simulink library "HvsOpen"  (Simulink 7.8)
settings: Solver=ode45  StartTime=0.0  StopTime=10.0  RelTol=1e-3
(part 1 of 2)
settings Model: Creator=KLJS168  LastModifiedBy=KLJS168

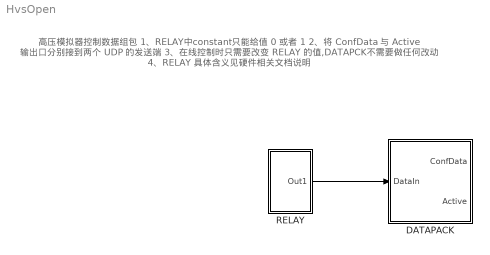
== system HvsOpen ==
  note: 高压模拟器控制数据组包
      | 1、RELAY中constant只能给值 0 或者 1
      | 2、将 ConfData 与 Active 输出口分别接到两个 UDP 的发送端
      | 3、在线控制时只需要改变 RELAY 的值,DATAPCK不需要做任何改动
      | 4、RELAY 具体含义见硬件相关文档说明
  DATAPACK : Subsystem
  RELAY : Subsystem
  wires:
  RELAY/1(Out1) -> DATAPACK/1(DataIn)

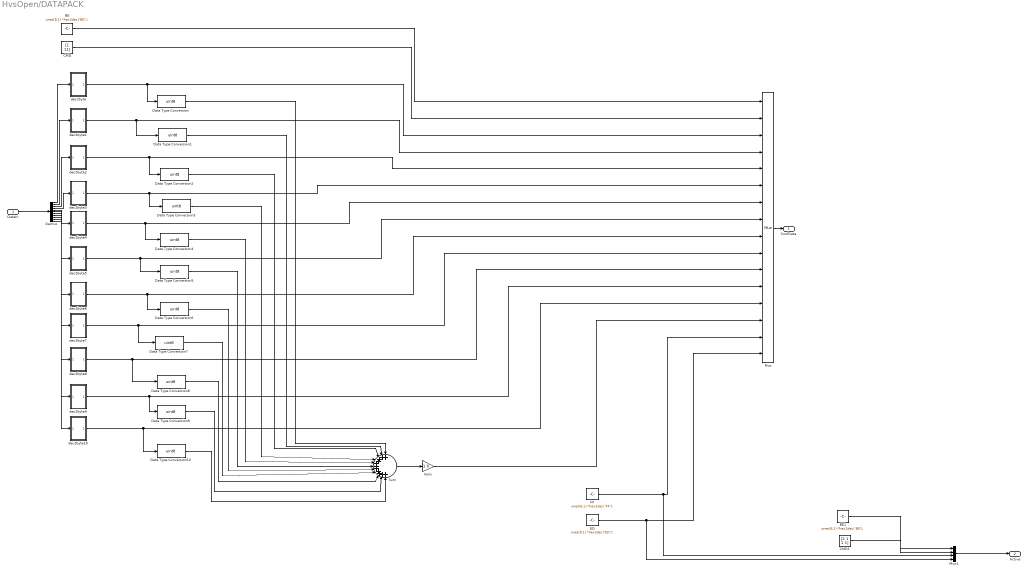
== system HvsOpen/DATAPACK ==
  DataIn : Inport
  BE : Constant  Value=ones(8,1).*hex2dec('BE');
  BE1 : Constant  Value=ones(8,1).*hex2dec('BE');
  CMD : Constant  Value=[1 11]
  CMD1 : Constant  Value=[2 1 1 1]
  Data Type Conversion{,1..10} (11 alike) : DataTypeConversion  OutDataTypeStr=uint8
  Demux : Demux  Outputs=[8 8 8 8 8 8 8 8 8 8 8]
  ED : Constant  Value=ones(8,1).*hex2dec('ED');
  FF : Constant  Value=ones(8,1).*hex2dec('FF');
  Gain : Gain  Gain=1.0  OutDataTypeStr=double
  Mux : Mux  Inputs=[8 2 1 1 1 1 1 1 1 1 1 1 1 1 8 8]
  Mux1 : Mux  Inputs=[8 4 8 8]
  Sum : Sum  Inputs=+++++++++++
  dec2byte : Subsystem
  dec2byte1 : Subsystem
  dec2byte10 : Subsystem
  dec2byte2 : Subsystem
  dec2byte3 : Subsystem
  dec2byte4 : Subsystem
  dec2byte5 : Subsystem
  dec2byte6 : Subsystem
  dec2byte7 : Subsystem
  dec2byte8 : Subsystem
  dec2byte9 : Subsystem
  ConfData : Outport
  Active : Outport  Port=2
  wires:
  BE/1 -> Mux/1
  CMD/1 -> Mux/2
  dec2byte/1(Out1) -> Mux/3, Data Type Conversion/1
  dec2byte1/1(Out1) -> Mux/4, Data Type Conversion1/1
  dec2byte2/1(Out1) -> Mux/5, Data Type Conversion2/1
  dec2byte3/1(Out1) -> Mux/6, Data Type Conversion3/1
  dec2byte4/1(Out1) -> Mux/7, Data Type Conversion4/1
  dec2byte5/1(Out1) -> Mux/8, Data Type Conversion5/1
  dec2byte6/1(Out1) -> Mux/9, Data Type Conversion6/1
  dec2byte7/1(Out1) -> Mux/10, Data Type Conversion7/1
  dec2byte8/1(Out1) -> Mux/11, Data Type Conversion8/1
  dec2byte9/1(Out1) -> Mux/12, Data Type Conversion9/1
  dec2byte10/1(Out1) -> Mux/13, Data Type Conversion10/1
  Sum/1 -> Gain/1
  Gain/1 -> Mux/14
  FF/1 -> Mux/15, Mux1/3
  ED/1 -> Mux/16, Mux1/4
  Data Type Conversion/1 -> Sum/1
  Data Type Conversion1/1 -> Sum/2
  Data Type Conversion2/1 -> Sum/3
  Data Type Conversion3/1 -> Sum/4
  Data Type Conversion4/1 -> Sum/5
  Data Type Conversion5/1 -> Sum/6
  Data Type Conversion6/1 -> Sum/7
  Data Type Conversion7/1 -> Sum/8
  Data Type Conversion8/1 -> Sum/9
  Data Type Conversion9/1 -> Sum/10
  Data Type Conversion10/1 -> Sum/11
  Mux/1 -> ConfData/1
  Demux/1 -> dec2byte/1(In1)
  Demux/2 -> dec2byte1/1(In1)
  Demux/3 -> dec2byte2/1(In1)
  Demux/4 -> dec2byte3/1(In1)
  Demux/5 -> dec2byte4/1(In1)
  Demux/6 -> dec2byte5/1(In1)
  Demux/7 -> dec2byte6/1(In1)
  Demux/8 -> dec2byte7/1(In1)
  Demux/9 -> dec2byte8/1(In1)
  Demux/10 -> dec2byte9/1(In1)
  Demux/11 -> dec2byte10/1(In1)
  DataIn/1 -> Demux/1
  BE1/1 -> Mux1/1
  CMD1/1 -> Mux1/2
  Mux1/1 -> Active/1

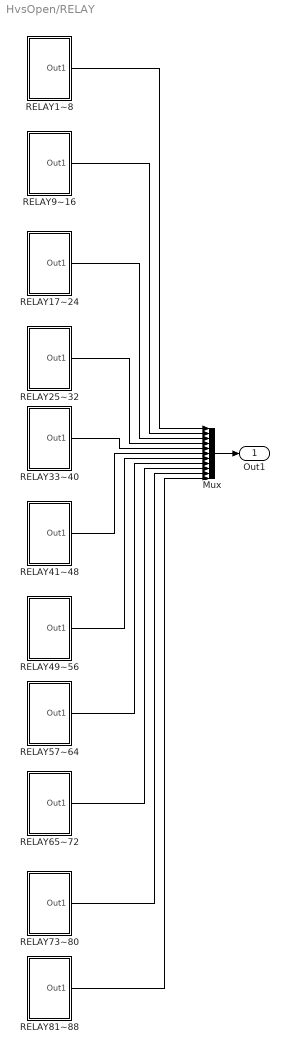
== system HvsOpen/RELAY ==
  Mux : Mux  Inputs=[8 8 8 8 8 8 8 8 8 8 8]
  RELAY17~24 : Subsystem
  RELAY1~8 : Subsystem
  RELAY25~32 : Subsystem
  RELAY33~40 : Subsystem
  RELAY41~48 : Subsystem
  RELAY49~56 : Subsystem
  RELAY57~64 : Subsystem
  RELAY65~72 : Subsystem
  RELAY73~80 : Subsystem
  RELAY81~88 : Subsystem
  RELAY9~16 : Subsystem
  Out1 : Outport
  wires:
  RELAY1~8/1(Out1) -> Mux/1
  RELAY9~16/1(Out1) -> Mux/2
  RELAY17~24/1(Out1) -> Mux/3
  RELAY25~32/1(Out1) -> Mux/4
  RELAY33~40/1(Out1) -> Mux/5
  RELAY41~48/1(Out1) -> Mux/6
  RELAY49~56/1(Out1) -> Mux/7
  RELAY57~64/1(Out1) -> Mux/8
  RELAY65~72/1(Out1) -> Mux/9
  RELAY73~80/1(Out1) -> Mux/10
  RELAY81~88/1(Out1) -> Mux/11
  Mux/1 -> Out1/1

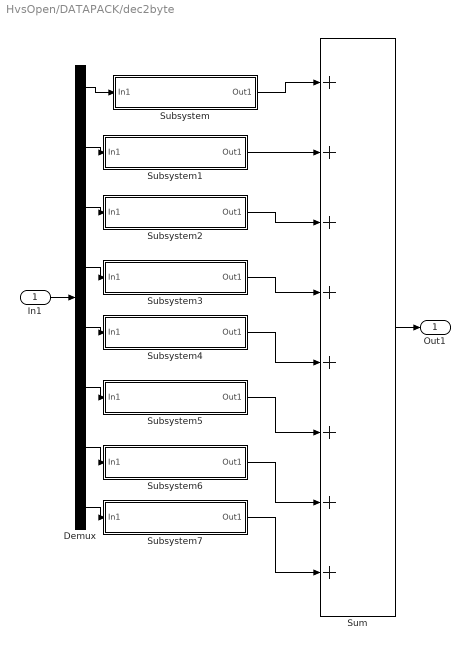
== system HvsOpen/DATAPACK/dec2byte ==
  In1 : Inport
  Demux : Demux  Outputs=8
  Subsystem : Subsystem  mask{power=0}
  Subsystem1 : Subsystem  mask{power=1}
  Subsystem2 : Subsystem  mask{power=2}
  Subsystem3 : Subsystem  mask{power=3}
  Subsystem4 : Subsystem  mask{power=4}
  Subsystem5 : Subsystem  mask{power=5}
  Subsystem6 : Subsystem  mask{power=6}
  Subsystem7 : Subsystem  mask{power=7}
  Sum : Sum  Inputs=++++++++
  Out1 : Outport
  wires:
  Demux/1 -> Subsystem/1(In1)
  Demux/2 -> Subsystem1/1(In1)
  Demux/3 -> Subsystem2/1(In1)
  Demux/4 -> Subsystem3/1(In1)
  Demux/5 -> Subsystem4/1(In1)
  Demux/6 -> Subsystem5/1(In1)
  Demux/7 -> Subsystem6/1(In1)
  Demux/8 -> Subsystem7/1(In1)
  Subsystem/1(Out1) -> Sum/1
  Subsystem1/1(Out1) -> Sum/2
  Subsystem2/1(Out1) -> Sum/3
  Subsystem3/1(Out1) -> Sum/4
  Subsystem4/1(Out1) -> Sum/5
  Subsystem5/1(Out1) -> Sum/6
  Subsystem6/1(Out1) -> Sum/7
  Subsystem7/1(Out1) -> Sum/8
  In1/1 -> Demux/1
  Sum/1 -> Out1/1

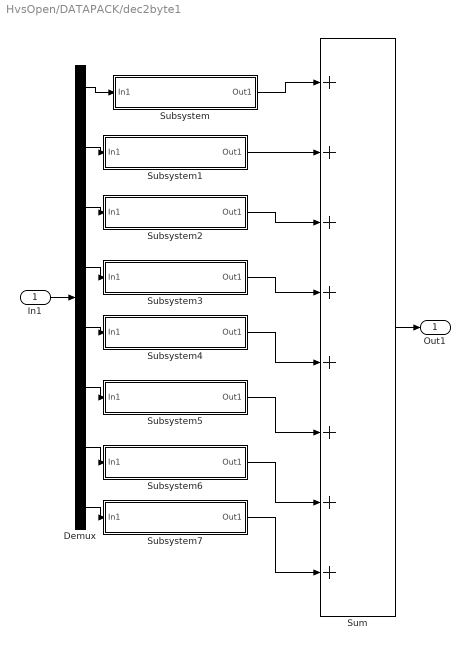
== system HvsOpen/DATAPACK/dec2byte1 ==
  In1 : Inport
  Demux : Demux  Outputs=8
  Subsystem : Subsystem  mask{power=0}
  Subsystem1 : Subsystem  mask{power=1}
  Subsystem2 : Subsystem  mask{power=2}
  Subsystem3 : Subsystem  mask{power=3}
  Subsystem4 : Subsystem  mask{power=4}
  Subsystem5 : Subsystem  mask{power=5}
  Subsystem6 : Subsystem  mask{power=6}
  Subsystem7 : Subsystem  mask{power=7}
  Sum : Sum  Inputs=++++++++
  Out1 : Outport
  wires:
  Sum/1 -> Out1/1
  In1/1 -> Demux/1
  Subsystem7/1(Out1) -> Sum/8
  Subsystem6/1(Out1) -> Sum/7
  Subsystem5/1(Out1) -> Sum/6
  Subsystem4/1(Out1) -> Sum/5
  Subsystem3/1(Out1) -> Sum/4
  Subsystem2/1(Out1) -> Sum/3
  Subsystem1/1(Out1) -> Sum/2
  Subsystem/1(Out1) -> Sum/1
  Demux/8 -> Subsystem7/1(In1)
  Demux/7 -> Subsystem6/1(In1)
  Demux/6 -> Subsystem5/1(In1)
  Demux/5 -> Subsystem4/1(In1)
  Demux/4 -> Subsystem3/1(In1)
  Demux/3 -> Subsystem2/1(In1)
  Demux/2 -> Subsystem1/1(In1)
  Demux/1 -> Subsystem/1(In1)

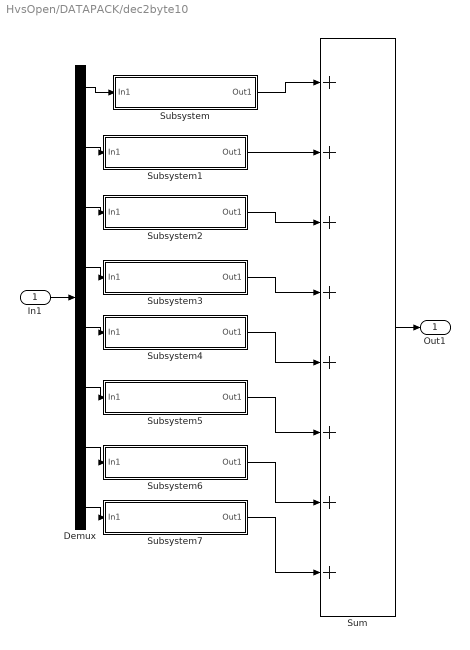
== system HvsOpen/DATAPACK/dec2byte10 ==
  In1 : Inport
  Demux : Demux  Outputs=8
  Subsystem : Subsystem  mask{power=0}
  Subsystem1 : Subsystem  mask{power=1}
  Subsystem2 : Subsystem  mask{power=2}
  Subsystem3 : Subsystem  mask{power=3}
  Subsystem4 : Subsystem  mask{power=4}
  Subsystem5 : Subsystem  mask{power=5}
  Subsystem6 : Subsystem  mask{power=6}
  Subsystem7 : Subsystem  mask{power=7}
  Sum : Sum  Inputs=++++++++
  Out1 : Outport
  wires:
  Demux/1 -> Subsystem/1(In1)
  Demux/2 -> Subsystem1/1(In1)
  Demux/3 -> Subsystem2/1(In1)
  Demux/4 -> Subsystem3/1(In1)
  Demux/5 -> Subsystem4/1(In1)
  Demux/6 -> Subsystem5/1(In1)
  Demux/7 -> Subsystem6/1(In1)
  Demux/8 -> Subsystem7/1(In1)
  Subsystem/1(Out1) -> Sum/1
  Subsystem1/1(Out1) -> Sum/2
  Subsystem2/1(Out1) -> Sum/3
  Subsystem3/1(Out1) -> Sum/4
  Subsystem4/1(Out1) -> Sum/5
  Subsystem5/1(Out1) -> Sum/6
  Subsystem6/1(Out1) -> Sum/7
  Subsystem7/1(Out1) -> Sum/8
  In1/1 -> Demux/1
  Sum/1 -> Out1/1

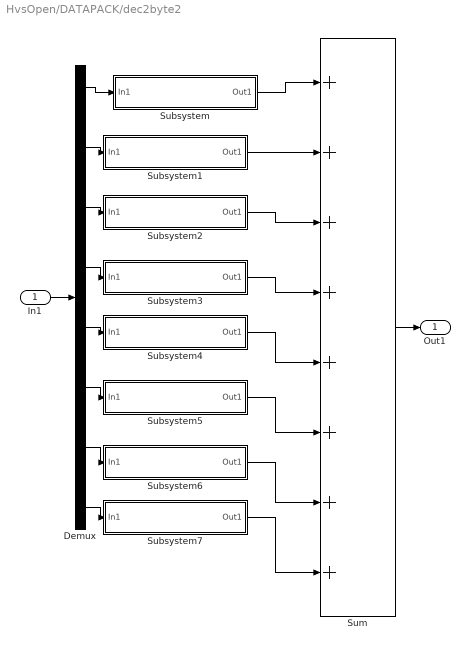
== system HvsOpen/DATAPACK/dec2byte2 ==
  In1 : Inport
  Demux : Demux  Outputs=8
  Subsystem : Subsystem  mask{power=0}
  Subsystem1 : Subsystem  mask{power=1}
  Subsystem2 : Subsystem  mask{power=2}
  Subsystem3 : Subsystem  mask{power=3}
  Subsystem4 : Subsystem  mask{power=4}
  Subsystem5 : Subsystem  mask{power=5}
  Subsystem6 : Subsystem  mask{power=6}
  Subsystem7 : Subsystem  mask{power=7}
  Sum : Sum  Inputs=++++++++
  Out1 : Outport
  wires:
  Demux/1 -> Subsystem/1(In1)
  Demux/2 -> Subsystem1/1(In1)
  Demux/3 -> Subsystem2/1(In1)
  Demux/4 -> Subsystem3/1(In1)
  Demux/5 -> Subsystem4/1(In1)
  Demux/6 -> Subsystem5/1(In1)
  Demux/7 -> Subsystem6/1(In1)
  Demux/8 -> Subsystem7/1(In1)
  Subsystem/1(Out1) -> Sum/1
  Subsystem1/1(Out1) -> Sum/2
  Subsystem2/1(Out1) -> Sum/3
  Subsystem3/1(Out1) -> Sum/4
  Subsystem4/1(Out1) -> Sum/5
  Subsystem5/1(Out1) -> Sum/6
  Subsystem6/1(Out1) -> Sum/7
  Subsystem7/1(Out1) -> Sum/8
  In1/1 -> Demux/1
  Sum/1 -> Out1/1

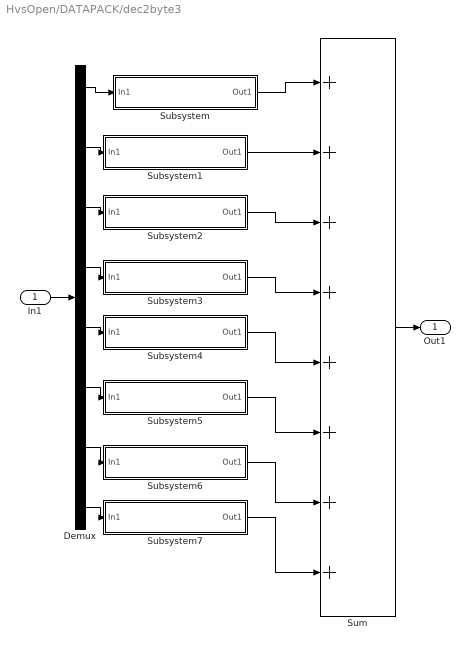
== system HvsOpen/DATAPACK/dec2byte3 ==
  In1 : Inport
  Demux : Demux  Outputs=8
  Subsystem : Subsystem  mask{power=0}
  Subsystem1 : Subsystem  mask{power=1}
  Subsystem2 : Subsystem  mask{power=2}
  Subsystem3 : Subsystem  mask{power=3}
  Subsystem4 : Subsystem  mask{power=4}
  Subsystem5 : Subsystem  mask{power=5}
  Subsystem6 : Subsystem  mask{power=6}
  Subsystem7 : Subsystem  mask{power=7}
  Sum : Sum  Inputs=++++++++
  Out1 : Outport
  wires:
  Sum/1 -> Out1/1
  In1/1 -> Demux/1
  Subsystem7/1(Out1) -> Sum/8
  Subsystem6/1(Out1) -> Sum/7
  Subsystem5/1(Out1) -> Sum/6
  Subsystem4/1(Out1) -> Sum/5
  Subsystem3/1(Out1) -> Sum/4
  Subsystem2/1(Out1) -> Sum/3
  Subsystem1/1(Out1) -> Sum/2
  Subsystem/1(Out1) -> Sum/1
  Demux/8 -> Subsystem7/1(In1)
  Demux/7 -> Subsystem6/1(In1)
  Demux/6 -> Subsystem5/1(In1)
  Demux/5 -> Subsystem4/1(In1)
  Demux/4 -> Subsystem3/1(In1)
  Demux/3 -> Subsystem2/1(In1)
  Demux/2 -> Subsystem1/1(In1)
  Demux/1 -> Subsystem/1(In1)

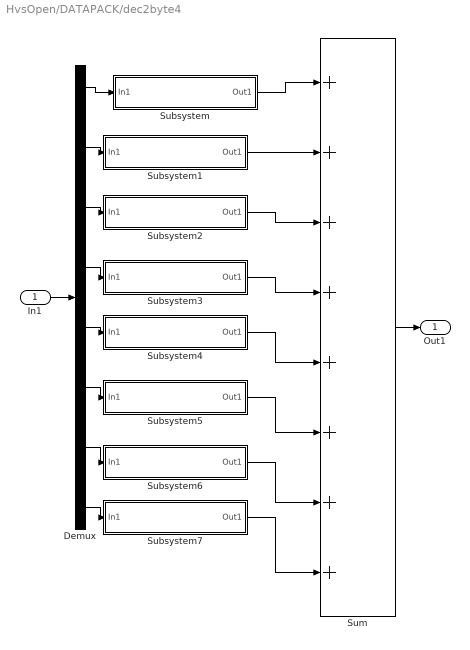
== system HvsOpen/DATAPACK/dec2byte4 ==
  In1 : Inport
  Demux : Demux  Outputs=8
  Subsystem : Subsystem  mask{power=0}
  Subsystem1 : Subsystem  mask{power=1}
  Subsystem2 : Subsystem  mask{power=2}
  Subsystem3 : Subsystem  mask{power=3}
  Subsystem4 : Subsystem  mask{power=4}
  Subsystem5 : Subsystem  mask{power=5}
  Subsystem6 : Subsystem  mask{power=6}
  Subsystem7 : Subsystem  mask{power=7}
  Sum : Sum  Inputs=++++++++
  Out1 : Outport
  wires:
  Demux/1 -> Subsystem/1(In1)
  Demux/2 -> Subsystem1/1(In1)
  Demux/3 -> Subsystem2/1(In1)
  Demux/4 -> Subsystem3/1(In1)
  Demux/5 -> Subsystem4/1(In1)
  Demux/6 -> Subsystem5/1(In1)
  Demux/7 -> Subsystem6/1(In1)
  Demux/8 -> Subsystem7/1(In1)
  Subsystem/1(Out1) -> Sum/1
  Subsystem1/1(Out1) -> Sum/2
  Subsystem2/1(Out1) -> Sum/3
  Subsystem3/1(Out1) -> Sum/4
  Subsystem4/1(Out1) -> Sum/5
  Subsystem5/1(Out1) -> Sum/6
  Subsystem6/1(Out1) -> Sum/7
  Subsystem7/1(Out1) -> Sum/8
  In1/1 -> Demux/1
  Sum/1 -> Out1/1

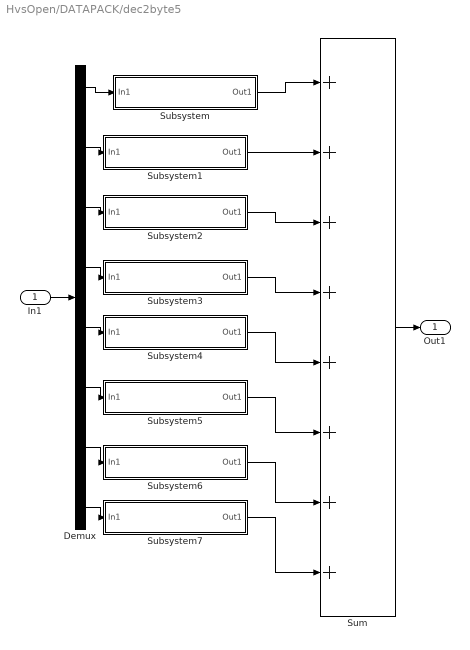
== system HvsOpen/DATAPACK/dec2byte5 ==
  In1 : Inport
  Demux : Demux  Outputs=8
  Subsystem : Subsystem  mask{power=0}
  Subsystem1 : Subsystem  mask{power=1}
  Subsystem2 : Subsystem  mask{power=2}
  Subsystem3 : Subsystem  mask{power=3}
  Subsystem4 : Subsystem  mask{power=4}
  Subsystem5 : Subsystem  mask{power=5}
  Subsystem6 : Subsystem  mask{power=6}
  Subsystem7 : Subsystem  mask{power=7}
  Sum : Sum  Inputs=++++++++
  Out1 : Outport
  wires:
  Sum/1 -> Out1/1
  In1/1 -> Demux/1
  Subsystem7/1(Out1) -> Sum/8
  Subsystem6/1(Out1) -> Sum/7
  Subsystem5/1(Out1) -> Sum/6
  Subsystem4/1(Out1) -> Sum/5
  Subsystem3/1(Out1) -> Sum/4
  Subsystem2/1(Out1) -> Sum/3
  Subsystem1/1(Out1) -> Sum/2
  Subsystem/1(Out1) -> Sum/1
  Demux/8 -> Subsystem7/1(In1)
  Demux/7 -> Subsystem6/1(In1)
  Demux/6 -> Subsystem5/1(In1)
  Demux/5 -> Subsystem4/1(In1)
  Demux/4 -> Subsystem3/1(In1)
  Demux/3 -> Subsystem2/1(In1)
  Demux/2 -> Subsystem1/1(In1)
  Demux/1 -> Subsystem/1(In1)

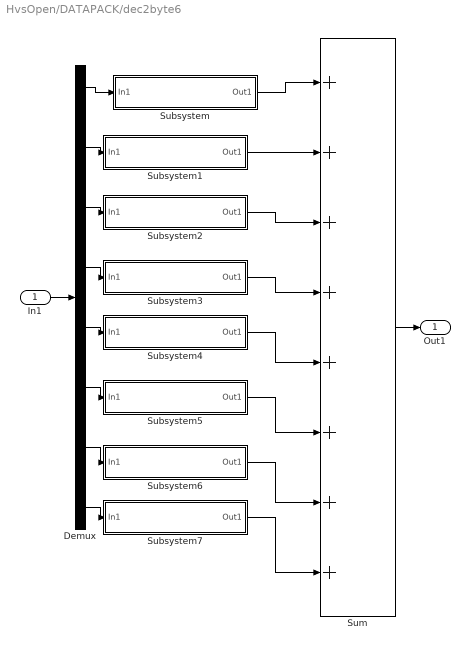
== system HvsOpen/DATAPACK/dec2byte6 ==
  In1 : Inport
  Demux : Demux  Outputs=8
  Subsystem : Subsystem  mask{power=0}
  Subsystem1 : Subsystem  mask{power=1}
  Subsystem2 : Subsystem  mask{power=2}
  Subsystem3 : Subsystem  mask{power=3}
  Subsystem4 : Subsystem  mask{power=4}
  Subsystem5 : Subsystem  mask{power=5}
  Subsystem6 : Subsystem  mask{power=6}
  Subsystem7 : Subsystem  mask{power=7}
  Sum : Sum  Inputs=++++++++
  Out1 : Outport
  wires:
  Demux/1 -> Subsystem/1(In1)
  Demux/2 -> Subsystem1/1(In1)
  Demux/3 -> Subsystem2/1(In1)
  Demux/4 -> Subsystem3/1(In1)
  Demux/5 -> Subsystem4/1(In1)
  Demux/6 -> Subsystem5/1(In1)
  Demux/7 -> Subsystem6/1(In1)
  Demux/8 -> Subsystem7/1(In1)
  Subsystem/1(Out1) -> Sum/1
  Subsystem1/1(Out1) -> Sum/2
  Subsystem2/1(Out1) -> Sum/3
  Subsystem3/1(Out1) -> Sum/4
  Subsystem4/1(Out1) -> Sum/5
  Subsystem5/1(Out1) -> Sum/6
  Subsystem6/1(Out1) -> Sum/7
  Subsystem7/1(Out1) -> Sum/8
  In1/1 -> Demux/1
  Sum/1 -> Out1/1

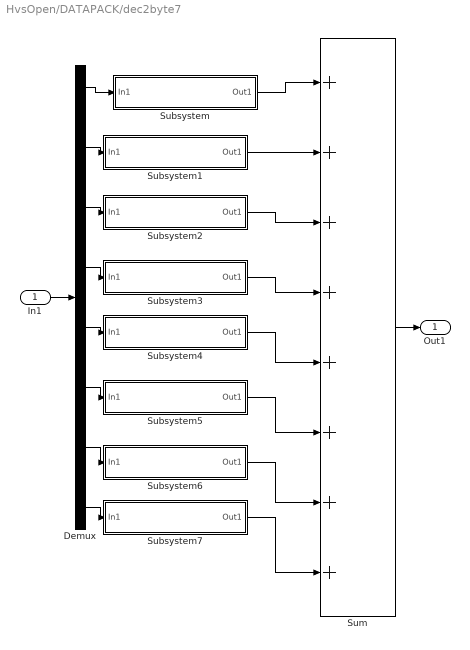
== system HvsOpen/DATAPACK/dec2byte7 ==
  In1 : Inport
  Demux : Demux  Outputs=8
  Subsystem : Subsystem  mask{power=0}
  Subsystem1 : Subsystem  mask{power=1}
  Subsystem2 : Subsystem  mask{power=2}
  Subsystem3 : Subsystem  mask{power=3}
  Subsystem4 : Subsystem  mask{power=4}
  Subsystem5 : Subsystem  mask{power=5}
  Subsystem6 : Subsystem  mask{power=6}
  Subsystem7 : Subsystem  mask{power=7}
  Sum : Sum  Inputs=++++++++
  Out1 : Outport
  wires:
  Sum/1 -> Out1/1
  In1/1 -> Demux/1
  Subsystem7/1(Out1) -> Sum/8
  Subsystem6/1(Out1) -> Sum/7
  Subsystem5/1(Out1) -> Sum/6
  Subsystem4/1(Out1) -> Sum/5
  Subsystem3/1(Out1) -> Sum/4
  Subsystem2/1(Out1) -> Sum/3
  Subsystem1/1(Out1) -> Sum/2
  Subsystem/1(Out1) -> Sum/1
  Demux/8 -> Subsystem7/1(In1)
  Demux/7 -> Subsystem6/1(In1)
  Demux/6 -> Subsystem5/1(In1)
  Demux/5 -> Subsystem4/1(In1)
  Demux/4 -> Subsystem3/1(In1)
  Demux/3 -> Subsystem2/1(In1)
  Demux/2 -> Subsystem1/1(In1)
  Demux/1 -> Subsystem/1(In1)

== system HvsOpen/DATAPACK/dec2byte8 ==
  In1 : Inport
  Demux : Demux  Outputs=8
  Subsystem : Subsystem  mask{power=0}
  Subsystem1 : Subsystem  mask{power=1}
  Subsystem2 : Subsystem  mask{power=2}
  Subsystem3 : Subsystem  mask{power=3}
  Subsystem4 : Subsystem  mask{power=4}
  Subsystem5 : Subsystem  mask{power=5}
  Subsystem6 : Subsystem  mask{power=6}
  Subsystem7 : Subsystem  mask{power=7}
  Sum : Sum  Inputs=++++++++
  Out1 : Outport
  wires:
  Demux/1 -> Subsystem/1(In1)
  Demux/2 -> Subsystem1/1(In1)
  Demux/3 -> Subsystem2/1(In1)
  Demux/4 -> Subsystem3/1(In1)
  Demux/5 -> Subsystem4/1(In1)
  Demux/6 -> Subsystem5/1(In1)
  Demux/7 -> Subsystem6/1(In1)
  Demux/8 -> Subsystem7/1(In1)
  Subsystem/1(Out1) -> Sum/1
  Subsystem1/1(Out1) -> Sum/2
  Subsystem2/1(Out1) -> Sum/3
  Subsystem3/1(Out1) -> Sum/4
  Subsystem4/1(Out1) -> Sum/5
  Subsystem5/1(Out1) -> Sum/6
  Subsystem6/1(Out1) -> Sum/7
  Subsystem7/1(Out1) -> Sum/8
  In1/1 -> Demux/1
  Sum/1 -> Out1/1

== system HvsOpen/DATAPACK/dec2byte9 ==
  In1 : Inport
  Demux : Demux  Outputs=8
  Subsystem : Subsystem  mask{power=0}
  Subsystem1 : Subsystem  mask{power=1}
  Subsystem2 : Subsystem  mask{power=2}
  Subsystem3 : Subsystem  mask{power=3}
  Subsystem4 : Subsystem  mask{power=4}
  Subsystem5 : Subsystem  mask{power=5}
  Subsystem6 : Subsystem  mask{power=6}
  Subsystem7 : Subsystem  mask{power=7}
  Sum : Sum  Inputs=++++++++
  Out1 : Outport
  wires:
  Sum/1 -> Out1/1
  In1/1 -> Demux/1
  Subsystem7/1(Out1) -> Sum/8
  Subsystem6/1(Out1) -> Sum/7
  Subsystem5/1(Out1) -> Sum/6
  Subsystem4/1(Out1) -> Sum/5
  Subsystem3/1(Out1) -> Sum/4
  Subsystem2/1(Out1) -> Sum/3
  Subsystem1/1(Out1) -> Sum/2
  Subsystem/1(Out1) -> Sum/1
  Demux/8 -> Subsystem7/1(In1)
  Demux/7 -> Subsystem6/1(In1)
  Demux/6 -> Subsystem5/1(In1)
  Demux/5 -> Subsystem4/1(In1)
  Demux/4 -> Subsystem3/1(In1)
  Demux/3 -> Subsystem2/1(In1)
  Demux/2 -> Subsystem1/1(In1)
  Demux/1 -> Subsystem/1(In1)

== system HvsOpen/RELAY/RELAY17~24 ==
  Mux : Mux  Inputs=8
  No USE : Constant  Value=0
  RELAY{18..24} (7 alike) : Constant  Value=0
  Out1 : Outport
  wires:
  Mux/1 -> Out1/1
  No USE/1 -> Mux/1
  RELAY18/1 -> Mux/2
  RELAY19/1 -> Mux/3
  RELAY20/1 -> Mux/4
  RELAY21/1 -> Mux/5
  RELAY22/1 -> Mux/6
  RELAY23/1 -> Mux/7
  RELAY24/1 -> Mux/8

== system HvsOpen/RELAY/RELAY1~8 ==
  Mux : Mux  Inputs=8
  RELAY{1..8} (8 alike) : Constant  Value=0
  Out1 : Outport
  wires:
  Mux/1 -> Out1/1
  RELAY1/1 -> Mux/1
  RELAY2/1 -> Mux/2
  RELAY3/1 -> Mux/3
  RELAY4/1 -> Mux/4
  RELAY5/1 -> Mux/5
  RELAY6/1 -> Mux/6
  RELAY7/1 -> Mux/7
  RELAY8/1 -> Mux/8

== system HvsOpen/RELAY/RELAY25~32 ==
  Mux : Mux  Inputs=8
  RELAY{25..32} (8 alike) : Constant  Value=0
  Out1 : Outport
  wires:
  RELAY32/1 -> Mux/8
  RELAY31/1 -> Mux/7
  RELAY30/1 -> Mux/6
  RELAY29/1 -> Mux/5
  RELAY28/1 -> Mux/4
  RELAY27/1 -> Mux/3
  RELAY26/1 -> Mux/2
  RELAY25/1 -> Mux/1
  Mux/1 -> Out1/1

== system HvsOpen/RELAY/RELAY33~40 ==
  Mux : Mux  Inputs=8
  RELAY{33..40} (8 alike) : Constant  Value=0
  Out1 : Outport
  wires:
  Mux/1 -> Out1/1
  RELAY33/1 -> Mux/1
  RELAY34/1 -> Mux/2
  RELAY35/1 -> Mux/3
  RELAY36/1 -> Mux/4
  RELAY37/1 -> Mux/5
  RELAY38/1 -> Mux/6
  RELAY39/1 -> Mux/7
  RELAY40/1 -> Mux/8

== system HvsOpen/RELAY/RELAY41~48 ==
  Mux : Mux  Inputs=8
  RELAY{41..48} (8 alike) : Constant  Value=0
  Out1 : Outport
  wires:
  RELAY48/1 -> Mux/8
  RELAY47/1 -> Mux/7
  RELAY46/1 -> Mux/6
  RELAY45/1 -> Mux/5
  RELAY44/1 -> Mux/4
  RELAY43/1 -> Mux/3
  RELAY42/1 -> Mux/2
  RELAY41/1 -> Mux/1
  Mux/1 -> Out1/1

== system HvsOpen/RELAY/RELAY49~56 ==
  Mux : Mux  Inputs=8
  RELAY{49..56} (8 alike) : Constant  Value=0
  Out1 : Outport
  wires:
  Mux/1 -> Out1/1
  RELAY49/1 -> Mux/1
  RELAY50/1 -> Mux/2
  RELAY51/1 -> Mux/3
  RELAY52/1 -> Mux/4
  RELAY53/1 -> Mux/5
  RELAY54/1 -> Mux/6
  RELAY55/1 -> Mux/7
  RELAY56/1 -> Mux/8

== system HvsOpen/RELAY/RELAY57~64 ==
  Mux : Mux  Inputs=8
  RELAY{57..64} (8 alike) : Constant  Value=0
  Out1 : Outport
  wires:
  RELAY64/1 -> Mux/8
  RELAY63/1 -> Mux/7
  RELAY62/1 -> Mux/6
  RELAY61/1 -> Mux/5
  RELAY60/1 -> Mux/4
  RELAY59/1 -> Mux/3
  RELAY58/1 -> Mux/2
  RELAY57/1 -> Mux/1
  Mux/1 -> Out1/1

== system HvsOpen/RELAY/RELAY65~72 ==
  Mux : Mux  Inputs=8
  RELAY{65..72} (8 alike) : Constant  Value=0
  Out1 : Outport
  wires:
  Mux/1 -> Out1/1
  RELAY65/1 -> Mux/1
  RELAY66/1 -> Mux/2
  RELAY67/1 -> Mux/3
  RELAY68/1 -> Mux/4
  RELAY69/1 -> Mux/5
  RELAY70/1 -> Mux/6
  RELAY71/1 -> Mux/7
  RELAY72/1 -> Mux/8

== system HvsOpen/RELAY/RELAY73~80 ==
  Mux : Mux  Inputs=8
  RELAY{73..80} (8 alike) : Constant  Value=0
  Out1 : Outport
  wires:
  RELAY80/1 -> Mux/8
  RELAY79/1 -> Mux/7
  RELAY78/1 -> Mux/6
  RELAY77/1 -> Mux/5
  RELAY76/1 -> Mux/4
  RELAY75/1 -> Mux/3
  RELAY74/1 -> Mux/2
  RELAY73/1 -> Mux/1
  Mux/1 -> Out1/1

== system HvsOpen/RELAY/RELAY81~88 ==
  Mux : Mux  Inputs=8
  No USE : Constant  Value=0
  No use : Constant  Value=0
  RELAY{81..86} (6 alike) : Constant  Value=0
  Out1 : Outport
  wires:
  Mux/1 -> Out1/1
  RELAY81/1 -> Mux/1
  RELAY82/1 -> Mux/2
  RELAY83/1 -> Mux/3
  RELAY84/1 -> Mux/4
  RELAY85/1 -> Mux/5
  RELAY86/1 -> Mux/6
  No USE/1 -> Mux/7
  No use/1 -> Mux/8

== system HvsOpen/RELAY/RELAY9~16 ==
  Mux : Mux  Inputs=8
  No use : Constant  Value=0
  No use1 : Constant  Value=0
  RELAY{9..13,16} (6 alike) : Constant  Value=0
  Out1 : Outport
  wires:
  Mux/1 -> Out1/1
  RELAY9/1 -> Mux/1
  RELAY10/1 -> Mux/2
  RELAY11/1 -> Mux/3
  RELAY12/1 -> Mux/4
  RELAY13/1 -> Mux/5
  No use/1 -> Mux/6
  No use1/1 -> Mux/7
  RELAY16/1 -> Mux/8

== system HvsOpen/DATAPACK/dec2byte/Subsystem ==
  In1 : Inport
  Constant8 : Constant  Value=power
  Constant9 : Constant  Value=2
  Math Function : Math  Operator=pow  SaturateOnIntegerOverflow=on
  Product : Product  RndMeth=Zero
  Out1 : Outport
  wires:
  Constant8/1 -> Math Function/2
  Constant9/1 -> Math Function/1
  Math Function/1 -> Product/2
  In1/1 -> Product/1
  Product/1 -> Out1/1

== system HvsOpen/DATAPACK/dec2byte/Subsystem1 ==
  In1 : Inport
  Constant8 : Constant  Value=power
  Constant9 : Constant  Value=2
  Math Function : Math  Operator=pow  SaturateOnIntegerOverflow=on
  Product : Product  RndMeth=Zero
  Out1 : Outport
  wires:
  Product/1 -> Out1/1
  In1/1 -> Product/1
  Math Function/1 -> Product/2
  Constant9/1 -> Math Function/1
  Constant8/1 -> Math Function/2

== system HvsOpen/DATAPACK/dec2byte/Subsystem2 ==
  In1 : Inport
  Constant8 : Constant  Value=power
  Constant9 : Constant  Value=2
  Math Function : Math  Operator=pow  SaturateOnIntegerOverflow=on
  Product : Product  RndMeth=Zero
  Out1 : Outport
  wires:
  Constant8/1 -> Math Function/2
  Constant9/1 -> Math Function/1
  Math Function/1 -> Product/2
  In1/1 -> Product/1
  Product/1 -> Out1/1

== system HvsOpen/DATAPACK/dec2byte/Subsystem3 ==
  In1 : Inport
  Constant8 : Constant  Value=power
  Constant9 : Constant  Value=2
  Math Function : Math  Operator=pow  SaturateOnIntegerOverflow=on
  Product : Product  RndMeth=Zero
  Out1 : Outport
  wires:
  Product/1 -> Out1/1
  In1/1 -> Product/1
  Math Function/1 -> Product/2
  Constant9/1 -> Math Function/1
  Constant8/1 -> Math Function/2

== system HvsOpen/DATAPACK/dec2byte/Subsystem4 ==
  In1 : Inport
  Constant8 : Constant  Value=power
  Constant9 : Constant  Value=2
  Math Function : Math  Operator=pow  SaturateOnIntegerOverflow=on
  Product : Product  RndMeth=Zero
  Out1 : Outport
  wires:
  Constant8/1 -> Math Function/2
  Constant9/1 -> Math Function/1
  Math Function/1 -> Product/2
  In1/1 -> Product/1
  Product/1 -> Out1/1

== system HvsOpen/DATAPACK/dec2byte/Subsystem5 ==
  In1 : Inport
  Constant8 : Constant  Value=power
  Constant9 : Constant  Value=2
  Math Function : Math  Operator=pow  SaturateOnIntegerOverflow=on
  Product : Product  RndMeth=Zero
  Out1 : Outport
  wires:
  Product/1 -> Out1/1
  In1/1 -> Product/1
  Math Function/1 -> Product/2
  Constant9/1 -> Math Function/1
  Constant8/1 -> Math Function/2

== system HvsOpen/DATAPACK/dec2byte/Subsystem6 ==
  In1 : Inport
  Constant8 : Constant  Value=power
  Constant9 : Constant  Value=2
  Math Function : Math  Operator=pow  SaturateOnIntegerOverflow=on
  Product : Product  RndMeth=Zero
  Out1 : Outport
  wires:
  Constant8/1 -> Math Function/2
  Constant9/1 -> Math Function/1
  Math Function/1 -> Product/2
  In1/1 -> Product/1
  Product/1 -> Out1/1

== system HvsOpen/DATAPACK/dec2byte/Subsystem7 ==
  In1 : Inport
  Constant8 : Constant  Value=power
  Constant9 : Constant  Value=2
  Math Function : Math  Operator=pow  SaturateOnIntegerOverflow=on
  Product : Product  RndMeth=Zero
  Out1 : Outport
  wires:
  Product/1 -> Out1/1
  In1/1 -> Product/1
  Math Function/1 -> Product/2
  Constant9/1 -> Math Function/1
  Constant8/1 -> Math Function/2

== system HvsOpen/DATAPACK/dec2byte1/Subsystem ==
  In1 : Inport
  Constant8 : Constant  Value=power
  Constant9 : Constant  Value=2
  Math Function : Math  Operator=pow  SaturateOnIntegerOverflow=on
  Product : Product  RndMeth=Zero
  Out1 : Outport
  wires:
  Product/1 -> Out1/1
  In1/1 -> Product/1
  Math Function/1 -> Product/2
  Constant9/1 -> Math Function/1
  Constant8/1 -> Math Function/2

== system HvsOpen/DATAPACK/dec2byte1/Subsystem1 ==
  In1 : Inport
  Constant8 : Constant  Value=power
  Constant9 : Constant  Value=2
  Math Function : Math  Operator=pow  SaturateOnIntegerOverflow=on
  Product : Product  RndMeth=Zero
  Out1 : Outport
  wires:
  Constant8/1 -> Math Function/2
  Constant9/1 -> Math Function/1
  Math Function/1 -> Product/2
  In1/1 -> Product/1
  Product/1 -> Out1/1

== system HvsOpen/DATAPACK/dec2byte1/Subsystem2 ==
  In1 : Inport
  Constant8 : Constant  Value=power
  Constant9 : Constant  Value=2
  Math Function : Math  Operator=pow  SaturateOnIntegerOverflow=on
  Product : Product  RndMeth=Zero
  Out1 : Outport
  wires:
  Product/1 -> Out1/1
  In1/1 -> Product/1
  Math Function/1 -> Product/2
  Constant9/1 -> Math Function/1
  Constant8/1 -> Math Function/2

== system HvsOpen/DATAPACK/dec2byte1/Subsystem3 ==
  In1 : Inport
  Constant8 : Constant  Value=power
  Constant9 : Constant  Value=2
  Math Function : Math  Operator=pow  SaturateOnIntegerOverflow=on
  Product : Product  RndMeth=Zero
  Out1 : Outport
  wires:
  Constant8/1 -> Math Function/2
  Constant9/1 -> Math Function/1
  Math Function/1 -> Product/2
  In1/1 -> Product/1
  Product/1 -> Out1/1

== system HvsOpen/DATAPACK/dec2byte1/Subsystem4 ==
  In1 : Inport
  Constant8 : Constant  Value=power
  Constant9 : Constant  Value=2
  Math Function : Math  Operator=pow  SaturateOnIntegerOverflow=on
  Product : Product  RndMeth=Zero
  Out1 : Outport
  wires:
  Product/1 -> Out1/1
  In1/1 -> Product/1
  Math Function/1 -> Product/2
  Constant9/1 -> Math Function/1
  Constant8/1 -> Math Function/2

== system HvsOpen/DATAPACK/dec2byte1/Subsystem5 ==
  In1 : Inport
  Constant8 : Constant  Value=power
  Constant9 : Constant  Value=2
  Math Function : Math  Operator=pow  SaturateOnIntegerOverflow=on
  Product : Product  RndMeth=Zero
  Out1 : Outport
  wires:
  Constant8/1 -> Math Function/2
  Constant9/1 -> Math Function/1
  Math Function/1 -> Product/2
  In1/1 -> Product/1
  Product/1 -> Out1/1

== system HvsOpen/DATAPACK/dec2byte1/Subsystem6 ==
  In1 : Inport
  Constant8 : Constant  Value=power
  Constant9 : Constant  Value=2
  Math Function : Math  Operator=pow  SaturateOnIntegerOverflow=on
  Product : Product  RndMeth=Zero
  Out1 : Outport
  wires:
  Product/1 -> Out1/1
  In1/1 -> Product/1
  Math Function/1 -> Product/2
  Constant9/1 -> Math Function/1
  Constant8/1 -> Math Function/2

== system HvsOpen/DATAPACK/dec2byte1/Subsystem7 ==
  In1 : Inport
  Constant8 : Constant  Value=power
  Constant9 : Constant  Value=2
  Math Function : Math  Operator=pow  SaturateOnIntegerOverflow=on
  Product : Product  RndMeth=Zero
  Out1 : Outport
  wires:
  Constant8/1 -> Math Function/2
  Constant9/1 -> Math Function/1
  Math Function/1 -> Product/2
  In1/1 -> Product/1
  Product/1 -> Out1/1

== system HvsOpen/DATAPACK/dec2byte10/Subsystem ==
  In1 : Inport
  Constant8 : Constant  Value=power
  Constant9 : Constant  Value=2
  Math Function : Math  Operator=pow  SaturateOnIntegerOverflow=on
  Product : Product  RndMeth=Zero
  Out1 : Outport
  wires:
  Constant8/1 -> Math Function/2
  Constant9/1 -> Math Function/1
  Math Function/1 -> Product/2
  In1/1 -> Product/1
  Product/1 -> Out1/1

== system HvsOpen/DATAPACK/dec2byte10/Subsystem1 ==
  In1 : Inport
  Constant8 : Constant  Value=power
  Constant9 : Constant  Value=2
  Math Function : Math  Operator=pow  SaturateOnIntegerOverflow=on
  Product : Product  RndMeth=Zero
  Out1 : Outport
  wires:
  Product/1 -> Out1/1
  In1/1 -> Product/1
  Math Function/1 -> Product/2
  Constant9/1 -> Math Function/1
  Constant8/1 -> Math Function/2

== system HvsOpen/DATAPACK/dec2byte10/Subsystem2 ==
  In1 : Inport
  Constant8 : Constant  Value=power
  Constant9 : Constant  Value=2
  Math Function : Math  Operator=pow  SaturateOnIntegerOverflow=on
  Product : Product  RndMeth=Zero
  Out1 : Outport
  wires:
  Constant8/1 -> Math Function/2
  Constant9/1 -> Math Function/1
  Math Function/1 -> Product/2
  In1/1 -> Product/1
  Product/1 -> Out1/1

== system HvsOpen/DATAPACK/dec2byte10/Subsystem3 ==
  In1 : Inport
  Constant8 : Constant  Value=power
  Constant9 : Constant  Value=2
  Math Function : Math  Operator=pow  SaturateOnIntegerOverflow=on
  Product : Product  RndMeth=Zero
  Out1 : Outport
  wires:
  Product/1 -> Out1/1
  In1/1 -> Product/1
  Math Function/1 -> Product/2
  Constant9/1 -> Math Function/1
  Constant8/1 -> Math Function/2

== system HvsOpen/DATAPACK/dec2byte10/Subsystem4 ==
  In1 : Inport
  Constant8 : Constant  Value=power
  Constant9 : Constant  Value=2
  Math Function : Math  Operator=pow  SaturateOnIntegerOverflow=on
  Product : Product  RndMeth=Zero
  Out1 : Outport
  wires:
  Constant8/1 -> Math Function/2
  Constant9/1 -> Math Function/1
  Math Function/1 -> Product/2
  In1/1 -> Product/1
  Product/1 -> Out1/1

== system HvsOpen/DATAPACK/dec2byte10/Subsystem5 ==
  In1 : Inport
  Constant8 : Constant  Value=power
  Constant9 : Constant  Value=2
  Math Function : Math  Operator=pow  SaturateOnIntegerOverflow=on
  Product : Product  RndMeth=Zero
  Out1 : Outport
  wires:
  Product/1 -> Out1/1
  In1/1 -> Product/1
  Math Function/1 -> Product/2
  Constant9/1 -> Math Function/1
  Constant8/1 -> Math Function/2

== system HvsOpen/DATAPACK/dec2byte10/Subsystem6 ==
  In1 : Inport
  Constant8 : Constant  Value=power
  Constant9 : Constant  Value=2
  Math Function : Math  Operator=pow  SaturateOnIntegerOverflow=on
  Product : Product  RndMeth=Zero
  Out1 : Outport
  wires:
  Constant8/1 -> Math Function/2
  Constant9/1 -> Math Function/1
  Math Function/1 -> Product/2
  In1/1 -> Product/1
  Product/1 -> Out1/1

== system HvsOpen/DATAPACK/dec2byte10/Subsystem7 ==
  In1 : Inport
  Constant8 : Constant  Value=power
  Constant9 : Constant  Value=2
  Math Function : Math  Operator=pow  SaturateOnIntegerOverflow=on
  Product : Product  RndMeth=Zero
  Out1 : Outport
  wires:
  Product/1 -> Out1/1
  In1/1 -> Product/1
  Math Function/1 -> Product/2
  Constant9/1 -> Math Function/1
  Constant8/1 -> Math Function/2

== system HvsOpen/DATAPACK/dec2byte2/Subsystem ==
  In1 : Inport
  Constant8 : Constant  Value=power
  Constant9 : Constant  Value=2
  Math Function : Math  Operator=pow  SaturateOnIntegerOverflow=on
  Product : Product  RndMeth=Zero
  Out1 : Outport
  wires:
  Constant8/1 -> Math Function/2
  Constant9/1 -> Math Function/1
  Math Function/1 -> Product/2
  In1/1 -> Product/1
  Product/1 -> Out1/1

== system HvsOpen/DATAPACK/dec2byte2/Subsystem1 ==
  In1 : Inport
  Constant8 : Constant  Value=power
  Constant9 : Constant  Value=2
  Math Function : Math  Operator=pow  SaturateOnIntegerOverflow=on
  Product : Product  RndMeth=Zero
  Out1 : Outport
  wires:
  Product/1 -> Out1/1
  In1/1 -> Product/1
  Math Function/1 -> Product/2
  Constant9/1 -> Math Function/1
  Constant8/1 -> Math Function/2

== system HvsOpen/DATAPACK/dec2byte2/Subsystem2 ==
  In1 : Inport
  Constant8 : Constant  Value=power
  Constant9 : Constant  Value=2
  Math Function : Math  Operator=pow  SaturateOnIntegerOverflow=on
  Product : Product  RndMeth=Zero
  Out1 : Outport
  wires:
  Constant8/1 -> Math Function/2
  Constant9/1 -> Math Function/1
  Math Function/1 -> Product/2
  In1/1 -> Product/1
  Product/1 -> Out1/1

== system HvsOpen/DATAPACK/dec2byte2/Subsystem3 ==
  In1 : Inport
  Constant8 : Constant  Value=power
  Constant9 : Constant  Value=2
  Math Function : Math  Operator=pow  SaturateOnIntegerOverflow=on
  Product : Product  RndMeth=Zero
  Out1 : Outport
  wires:
  Product/1 -> Out1/1
  In1/1 -> Product/1
  Math Function/1 -> Product/2
  Constant9/1 -> Math Function/1
  Constant8/1 -> Math Function/2

== system HvsOpen/DATAPACK/dec2byte2/Subsystem4 ==
  In1 : Inport
  Constant8 : Constant  Value=power
  Constant9 : Constant  Value=2
  Math Function : Math  Operator=pow  SaturateOnIntegerOverflow=on
  Product : Product  RndMeth=Zero
  Out1 : Outport
  wires:
  Constant8/1 -> Math Function/2
  Constant9/1 -> Math Function/1
  Math Function/1 -> Product/2
  In1/1 -> Product/1
  Product/1 -> Out1/1

== system HvsOpen/DATAPACK/dec2byte2/Subsystem5 ==
  In1 : Inport
  Constant8 : Constant  Value=power
  Constant9 : Constant  Value=2
  Math Function : Math  Operator=pow  SaturateOnIntegerOverflow=on
  Product : Product  RndMeth=Zero
  Out1 : Outport
  wires:
  Product/1 -> Out1/1
  In1/1 -> Product/1
  Math Function/1 -> Product/2
  Constant9/1 -> Math Function/1
  Constant8/1 -> Math Function/2

== system HvsOpen/DATAPACK/dec2byte2/Subsystem6 ==
  In1 : Inport
  Constant8 : Constant  Value=power
  Constant9 : Constant  Value=2
  Math Function : Math  Operator=pow  SaturateOnIntegerOverflow=on
  Product : Product  RndMeth=Zero
  Out1 : Outport
  wires:
  Constant8/1 -> Math Function/2
  Constant9/1 -> Math Function/1
  Math Function/1 -> Product/2
  In1/1 -> Product/1
  Product/1 -> Out1/1

== system HvsOpen/DATAPACK/dec2byte2/Subsystem7 ==
  In1 : Inport
  Constant8 : Constant  Value=power
  Constant9 : Constant  Value=2
  Math Function : Math  Operator=pow  SaturateOnIntegerOverflow=on
  Product : Product  RndMeth=Zero
  Out1 : Outport
  wires:
  Product/1 -> Out1/1
  In1/1 -> Product/1
  Math Function/1 -> Product/2
  Constant9/1 -> Math Function/1
  Constant8/1 -> Math Function/2

== system HvsOpen/DATAPACK/dec2byte3/Subsystem ==
  In1 : Inport
  Constant8 : Constant  Value=power
  Constant9 : Constant  Value=2
  Math Function : Math  Operator=pow  SaturateOnIntegerOverflow=on
  Product : Product  RndMeth=Zero
  Out1 : Outport
  wires:
  Product/1 -> Out1/1
  In1/1 -> Product/1
  Math Function/1 -> Product/2
  Constant9/1 -> Math Function/1
  Constant8/1 -> Math Function/2

== system HvsOpen/DATAPACK/dec2byte3/Subsystem1 ==
  In1 : Inport
  Constant8 : Constant  Value=power
  Constant9 : Constant  Value=2
  Math Function : Math  Operator=pow  SaturateOnIntegerOverflow=on
  Product : Product  RndMeth=Zero
  Out1 : Outport
  wires:
  Constant8/1 -> Math Function/2
  Constant9/1 -> Math Function/1
  Math Function/1 -> Product/2
  In1/1 -> Product/1
  Product/1 -> Out1/1

== system HvsOpen/DATAPACK/dec2byte3/Subsystem2 ==
  In1 : Inport
  Constant8 : Constant  Value=power
  Constant9 : Constant  Value=2
  Math Function : Math  Operator=pow  SaturateOnIntegerOverflow=on
  Product : Product  RndMeth=Zero
  Out1 : Outport
  wires:
  Product/1 -> Out1/1
  In1/1 -> Product/1
  Math Function/1 -> Product/2
  Constant9/1 -> Math Function/1
  Constant8/1 -> Math Function/2

== system HvsOpen/DATAPACK/dec2byte3/Subsystem3 ==
  In1 : Inport
  Constant8 : Constant  Value=power
  Constant9 : Constant  Value=2
  Math Function : Math  Operator=pow  SaturateOnIntegerOverflow=on
  Product : Product  RndMeth=Zero
  Out1 : Outport
  wires:
  Constant8/1 -> Math Function/2
  Constant9/1 -> Math Function/1
  Math Function/1 -> Product/2
  In1/1 -> Product/1
  Product/1 -> Out1/1

== system HvsOpen/DATAPACK/dec2byte3/Subsystem4 ==
  In1 : Inport
  Constant8 : Constant  Value=power
  Constant9 : Constant  Value=2
  Math Function : Math  Operator=pow  SaturateOnIntegerOverflow=on
  Product : Product  RndMeth=Zero
  Out1 : Outport
  wires:
  Product/1 -> Out1/1
  In1/1 -> Product/1
  Math Function/1 -> Product/2
  Constant9/1 -> Math Function/1
  Constant8/1 -> Math Function/2

== system HvsOpen/DATAPACK/dec2byte3/Subsystem5 ==
  In1 : Inport
  Constant8 : Constant  Value=power
  Constant9 : Constant  Value=2
  Math Function : Math  Operator=pow  SaturateOnIntegerOverflow=on
  Product : Product  RndMeth=Zero
  Out1 : Outport
  wires:
  Constant8/1 -> Math Function/2
  Constant9/1 -> Math Function/1
  Math Function/1 -> Product/2
  In1/1 -> Product/1
  Product/1 -> Out1/1

== system HvsOpen/DATAPACK/dec2byte3/Subsystem6 ==
  In1 : Inport
  Constant8 : Constant  Value=power
  Constant9 : Constant  Value=2
  Math Function : Math  Operator=pow  SaturateOnIntegerOverflow=on
  Product : Product  RndMeth=Zero
  Out1 : Outport
  wires:
  Product/1 -> Out1/1
  In1/1 -> Product/1
  Math Function/1 -> Product/2
  Constant9/1 -> Math Function/1
  Constant8/1 -> Math Function/2

== system HvsOpen/DATAPACK/dec2byte3/Subsystem7 ==
  In1 : Inport
  Constant8 : Constant  Value=power
  Constant9 : Constant  Value=2
  Math Function : Math  Operator=pow  SaturateOnIntegerOverflow=on
  Product : Product  RndMeth=Zero
  Out1 : Outport
  wires:
  Constant8/1 -> Math Function/2
  Constant9/1 -> Math Function/1
  Math Function/1 -> Product/2
  In1/1 -> Product/1
  Product/1 -> Out1/1

== system HvsOpen/DATAPACK/dec2byte4/Subsystem ==
  In1 : Inport
  Constant8 : Constant  Value=power
  Constant9 : Constant  Value=2
  Math Function : Math  Operator=pow  SaturateOnIntegerOverflow=on
  Product : Product  RndMeth=Zero
  Out1 : Outport
  wires:
  Constant8/1 -> Math Function/2
  Constant9/1 -> Math Function/1
  Math Function/1 -> Product/2
  In1/1 -> Product/1
  Product/1 -> Out1/1

== system HvsOpen/DATAPACK/dec2byte4/Subsystem1 ==
  In1 : Inport
  Constant8 : Constant  Value=power
  Constant9 : Constant  Value=2
  Math Function : Math  Operator=pow  SaturateOnIntegerOverflow=on
  Product : Product  RndMeth=Zero
  Out1 : Outport
  wires:
  Product/1 -> Out1/1
  In1/1 -> Product/1
  Math Function/1 -> Product/2
  Constant9/1 -> Math Function/1
  Constant8/1 -> Math Function/2

== system HvsOpen/DATAPACK/dec2byte4/Subsystem2 ==
  In1 : Inport
  Constant8 : Constant  Value=power
  Constant9 : Constant  Value=2
  Math Function : Math  Operator=pow  SaturateOnIntegerOverflow=on
  Product : Product  RndMeth=Zero
  Out1 : Outport
  wires:
  Constant8/1 -> Math Function/2
  Constant9/1 -> Math Function/1
  Math Function/1 -> Product/2
  In1/1 -> Product/1
  Product/1 -> Out1/1

== system HvsOpen/DATAPACK/dec2byte4/Subsystem3 ==
  In1 : Inport
  Constant8 : Constant  Value=power
  Constant9 : Constant  Value=2
  Math Function : Math  Operator=pow  SaturateOnIntegerOverflow=on
  Product : Product  RndMeth=Zero
  Out1 : Outport
  wires:
  Product/1 -> Out1/1
  In1/1 -> Product/1
  Math Function/1 -> Product/2
  Constant9/1 -> Math Function/1
  Constant8/1 -> Math Function/2

== system HvsOpen/DATAPACK/dec2byte4/Subsystem4 ==
  In1 : Inport
  Constant8 : Constant  Value=power
  Constant9 : Constant  Value=2
  Math Function : Math  Operator=pow  SaturateOnIntegerOverflow=on
  Product : Product  RndMeth=Zero
  Out1 : Outport
  wires:
  Constant8/1 -> Math Function/2
  Constant9/1 -> Math Function/1
  Math Function/1 -> Product/2
  In1/1 -> Product/1
  Product/1 -> Out1/1

== system HvsOpen/DATAPACK/dec2byte4/Subsystem5 ==
  In1 : Inport
  Constant8 : Constant  Value=power
  Constant9 : Constant  Value=2
  Math Function : Math  Operator=pow  SaturateOnIntegerOverflow=on
  Product : Product  RndMeth=Zero
  Out1 : Outport
  wires:
  Product/1 -> Out1/1
  In1/1 -> Product/1
  Math Function/1 -> Product/2
  Constant9/1 -> Math Function/1
  Constant8/1 -> Math Function/2

== system HvsOpen/DATAPACK/dec2byte4/Subsystem6 ==
  In1 : Inport
  Constant8 : Constant  Value=power
  Constant9 : Constant  Value=2
  Math Function : Math  Operator=pow  SaturateOnIntegerOverflow=on
  Product : Product  RndMeth=Zero
  Out1 : Outport
  wires:
  Constant8/1 -> Math Function/2
  Constant9/1 -> Math Function/1
  Math Function/1 -> Product/2
  In1/1 -> Product/1
  Product/1 -> Out1/1

== system HvsOpen/DATAPACK/dec2byte4/Subsystem7 ==
  In1 : Inport
  Constant8 : Constant  Value=power
  Constant9 : Constant  Value=2
  Math Function : Math  Operator=pow  SaturateOnIntegerOverflow=on
  Product : Product  RndMeth=Zero
  Out1 : Outport
  wires:
  Product/1 -> Out1/1
  In1/1 -> Product/1
  Math Function/1 -> Product/2
  Constant9/1 -> Math Function/1
  Constant8/1 -> Math Function/2

== system HvsOpen/DATAPACK/dec2byte5/Subsystem ==
  In1 : Inport
  Constant8 : Constant  Value=power
  Constant9 : Constant  Value=2
  Math Function : Math  Operator=pow  SaturateOnIntegerOverflow=on
  Product : Product  RndMeth=Zero
  Out1 : Outport
  wires:
  Product/1 -> Out1/1
  In1/1 -> Product/1
  Math Function/1 -> Product/2
  Constant9/1 -> Math Function/1
  Constant8/1 -> Math Function/2

== system HvsOpen/DATAPACK/dec2byte5/Subsystem1 ==
  In1 : Inport
  Constant8 : Constant  Value=power
  Constant9 : Constant  Value=2
  Math Function : Math  Operator=pow  SaturateOnIntegerOverflow=on
  Product : Product  RndMeth=Zero
  Out1 : Outport
  wires:
  Constant8/1 -> Math Function/2
  Constant9/1 -> Math Function/1
  Math Function/1 -> Product/2
  In1/1 -> Product/1
  Product/1 -> Out1/1

== system HvsOpen/DATAPACK/dec2byte5/Subsystem2 ==
  In1 : Inport
  Constant8 : Constant  Value=power
  Constant9 : Constant  Value=2
  Math Function : Math  Operator=pow  SaturateOnIntegerOverflow=on
  Product : Product  RndMeth=Zero
  Out1 : Outport
  wires:
  Product/1 -> Out1/1
  In1/1 -> Product/1
  Math Function/1 -> Product/2
  Constant9/1 -> Math Function/1
  Constant8/1 -> Math Function/2

== system HvsOpen/DATAPACK/dec2byte5/Subsystem3 ==
  In1 : Inport
  Constant8 : Constant  Value=power
  Constant9 : Constant  Value=2
  Math Function : Math  Operator=pow  SaturateOnIntegerOverflow=on
  Product : Product  RndMeth=Zero
  Out1 : Outport
  wires:
  Constant8/1 -> Math Function/2
  Constant9/1 -> Math Function/1
  Math Function/1 -> Product/2
  In1/1 -> Product/1
  Product/1 -> Out1/1

== system HvsOpen/DATAPACK/dec2byte5/Subsystem4 ==
  In1 : Inport
  Constant8 : Constant  Value=power
  Constant9 : Constant  Value=2
  Math Function : Math  Operator=pow  SaturateOnIntegerOverflow=on
  Product : Product  RndMeth=Zero
  Out1 : Outport
  wires:
  Product/1 -> Out1/1
  In1/1 -> Product/1
  Math Function/1 -> Product/2
  Constant9/1 -> Math Function/1
  Constant8/1 -> Math Function/2

== system HvsOpen/DATAPACK/dec2byte5/Subsystem5 ==
  In1 : Inport
  Constant8 : Constant  Value=power
  Constant9 : Constant  Value=2
  Math Function : Math  Operator=pow  SaturateOnIntegerOverflow=on
  Product : Product  RndMeth=Zero
  Out1 : Outport
  wires:
  Constant8/1 -> Math Function/2
  Constant9/1 -> Math Function/1
  Math Function/1 -> Product/2
  In1/1 -> Product/1
  Product/1 -> Out1/1

== system HvsOpen/DATAPACK/dec2byte5/Subsystem6 ==
  In1 : Inport
  Constant8 : Constant  Value=power
  Constant9 : Constant  Value=2
  Math Function : Math  Operator=pow  SaturateOnIntegerOverflow=on
  Product : Product  RndMeth=Zero
  Out1 : Outport
  wires:
  Product/1 -> Out1/1
  In1/1 -> Product/1
  Math Function/1 -> Product/2
  Constant9/1 -> Math Function/1
  Constant8/1 -> Math Function/2

== system HvsOpen/DATAPACK/dec2byte5/Subsystem7 ==
  In1 : Inport
  Constant8 : Constant  Value=power
  Constant9 : Constant  Value=2
  Math Function : Math  Operator=pow  SaturateOnIntegerOverflow=on
  Product : Product  RndMeth=Zero
  Out1 : Outport
  wires:
  Constant8/1 -> Math Function/2
  Constant9/1 -> Math Function/1
  Math Function/1 -> Product/2
  In1/1 -> Product/1
  Product/1 -> Out1/1

== system HvsOpen/DATAPACK/dec2byte6/Subsystem ==
  In1 : Inport
  Constant8 : Constant  Value=power
  Constant9 : Constant  Value=2
  Math Function : Math  Operator=pow  SaturateOnIntegerOverflow=on
  Product : Product  RndMeth=Zero
  Out1 : Outport
  wires:
  Constant8/1 -> Math Function/2
  Constant9/1 -> Math Function/1
  Math Function/1 -> Product/2
  In1/1 -> Product/1
  Product/1 -> Out1/1

== system HvsOpen/DATAPACK/dec2byte6/Subsystem1 ==
  In1 : Inport
  Constant8 : Constant  Value=power
  Constant9 : Constant  Value=2
  Math Function : Math  Operator=pow  SaturateOnIntegerOverflow=on
  Product : Product  RndMeth=Zero
  Out1 : Outport
  wires:
  Product/1 -> Out1/1
  In1/1 -> Product/1
  Math Function/1 -> Product/2
  Constant9/1 -> Math Function/1
  Constant8/1 -> Math Function/2

== system HvsOpen/DATAPACK/dec2byte6/Subsystem2 ==
  In1 : Inport
  Constant8 : Constant  Value=power
  Constant9 : Constant  Value=2
  Math Function : Math  Operator=pow  SaturateOnIntegerOverflow=on
  Product : Product  RndMeth=Zero
  Out1 : Outport
  wires:
  Constant8/1 -> Math Function/2
  Constant9/1 -> Math Function/1
  Math Function/1 -> Product/2
  In1/1 -> Product/1
  Product/1 -> Out1/1

== system HvsOpen/DATAPACK/dec2byte6/Subsystem3 ==
  In1 : Inport
  Constant8 : Constant  Value=power
  Constant9 : Constant  Value=2
  Math Function : Math  Operator=pow  SaturateOnIntegerOverflow=on
  Product : Product  RndMeth=Zero
  Out1 : Outport
  wires:
  Product/1 -> Out1/1
  In1/1 -> Product/1
  Math Function/1 -> Product/2
  Constant9/1 -> Math Function/1
  Constant8/1 -> Math Function/2

== system HvsOpen/DATAPACK/dec2byte6/Subsystem4 ==
  In1 : Inport
  Constant8 : Constant  Value=power
  Constant9 : Constant  Value=2
  Math Function : Math  Operator=pow  SaturateOnIntegerOverflow=on
  Product : Product  RndMeth=Zero
  Out1 : Outport
  wires:
  Constant8/1 -> Math Function/2
  Constant9/1 -> Math Function/1
  Math Function/1 -> Product/2
  In1/1 -> Product/1
  Product/1 -> Out1/1

== system HvsOpen/DATAPACK/dec2byte6/Subsystem5 ==
  In1 : Inport
  Constant8 : Constant  Value=power
  Constant9 : Constant  Value=2
  Math Function : Math  Operator=pow  SaturateOnIntegerOverflow=on
  Product : Product  RndMeth=Zero
  Out1 : Outport
  wires:
  Product/1 -> Out1/1
  In1/1 -> Product/1
  Math Function/1 -> Product/2
  Constant9/1 -> Math Function/1
  Constant8/1 -> Math Function/2

== system HvsOpen/DATAPACK/dec2byte6/Subsystem6 ==
  In1 : Inport
  Constant8 : Constant  Value=power
  Constant9 : Constant  Value=2
  Math Function : Math  Operator=pow  SaturateOnIntegerOverflow=on
  Product : Product  RndMeth=Zero
  Out1 : Outport
  wires:
  Constant8/1 -> Math Function/2
  Constant9/1 -> Math Function/1
  Math Function/1 -> Product/2
  In1/1 -> Product/1
  Product/1 -> Out1/1

== system HvsOpen/DATAPACK/dec2byte6/Subsystem7 ==
  In1 : Inport
  Constant8 : Constant  Value=power
  Constant9 : Constant  Value=2
  Math Function : Math  Operator=pow  SaturateOnIntegerOverflow=on
  Product : Product  RndMeth=Zero
  Out1 : Outport
  wires:
  Product/1 -> Out1/1
  In1/1 -> Product/1
  Math Function/1 -> Product/2
  Constant9/1 -> Math Function/1
  Constant8/1 -> Math Function/2

== system HvsOpen/DATAPACK/dec2byte7/Subsystem ==
  In1 : Inport
  Constant8 : Constant  Value=power
  Constant9 : Constant  Value=2
  Math Function : Math  Operator=pow  SaturateOnIntegerOverflow=on
  Product : Product  RndMeth=Zero
  Out1 : Outport
  wires:
  Product/1 -> Out1/1
  In1/1 -> Product/1
  Math Function/1 -> Product/2
  Constant9/1 -> Math Function/1
  Constant8/1 -> Math Function/2

== system HvsOpen/DATAPACK/dec2byte7/Subsystem1 ==
  In1 : Inport
  Constant8 : Constant  Value=power
  Constant9 : Constant  Value=2
  Math Function : Math  Operator=pow  SaturateOnIntegerOverflow=on
  Product : Product  RndMeth=Zero
  Out1 : Outport
  wires:
  Constant8/1 -> Math Function/2
  Constant9/1 -> Math Function/1
  Math Function/1 -> Product/2
  In1/1 -> Product/1
  Product/1 -> Out1/1

== system HvsOpen/DATAPACK/dec2byte7/Subsystem2 ==
  In1 : Inport
  Constant8 : Constant  Value=power
  Constant9 : Constant  Value=2
  Math Function : Math  Operator=pow  SaturateOnIntegerOverflow=on
  Product : Product  RndMeth=Zero
  Out1 : Outport
  wires:
  Product/1 -> Out1/1
  In1/1 -> Product/1
  Math Function/1 -> Product/2
  Constant9/1 -> Math Function/1
  Constant8/1 -> Math Function/2

== system HvsOpen/DATAPACK/dec2byte7/Subsystem3 ==
  In1 : Inport
  Constant8 : Constant  Value=power
  Constant9 : Constant  Value=2
  Math Function : Math  Operator=pow  SaturateOnIntegerOverflow=on
  Product : Product  RndMeth=Zero
  Out1 : Outport
  wires:
  Constant8/1 -> Math Function/2
  Constant9/1 -> Math Function/1
  Math Function/1 -> Product/2
  In1/1 -> Product/1
  Product/1 -> Out1/1

== system HvsOpen/DATAPACK/dec2byte7/Subsystem4 ==
  In1 : Inport
  Constant8 : Constant  Value=power
  Constant9 : Constant  Value=2
  Math Function : Math  Operator=pow  SaturateOnIntegerOverflow=on
  Product : Product  RndMeth=Zero
  Out1 : Outport
  wires:
  Product/1 -> Out1/1
  In1/1 -> Product/1
  Math Function/1 -> Product/2
  Constant9/1 -> Math Function/1
  Constant8/1 -> Math Function/2

== system HvsOpen/DATAPACK/dec2byte7/Subsystem5 ==
  In1 : Inport
  Constant8 : Constant  Value=power
  Constant9 : Constant  Value=2
  Math Function : Math  Operator=pow  SaturateOnIntegerOverflow=on
  Product : Product  RndMeth=Zero
  Out1 : Outport
  wires:
  Constant8/1 -> Math Function/2
  Constant9/1 -> Math Function/1
  Math Function/1 -> Product/2
  In1/1 -> Product/1
  Product/1 -> Out1/1

== system HvsOpen/DATAPACK/dec2byte7/Subsystem6 ==
  In1 : Inport
  Constant8 : Constant  Value=power
  Constant9 : Constant  Value=2
  Math Function : Math  Operator=pow  SaturateOnIntegerOverflow=on
  Product : Product  RndMeth=Zero
  Out1 : Outport
  wires:
  Product/1 -> Out1/1
  In1/1 -> Product/1
  Math Function/1 -> Product/2
  Constant9/1 -> Math Function/1
  Constant8/1 -> Math Function/2

== system HvsOpen/DATAPACK/dec2byte7/Subsystem7 ==
  In1 : Inport
  Constant8 : Constant  Value=power
  Constant9 : Constant  Value=2
  Math Function : Math  Operator=pow  SaturateOnIntegerOverflow=on
  Product : Product  RndMeth=Zero
  Out1 : Outport
  wires:
  Constant8/1 -> Math Function/2
  Constant9/1 -> Math Function/1
  Math Function/1 -> Product/2
  In1/1 -> Product/1
  Product/1 -> Out1/1

== system HvsOpen/DATAPACK/dec2byte8/Subsystem ==
  In1 : Inport
  Constant8 : Constant  Value=power
  Constant9 : Constant  Value=2
  Math Function : Math  Operator=pow  SaturateOnIntegerOverflow=on
  Product : Product  RndMeth=Zero
  Out1 : Outport
  wires:
  Constant8/1 -> Math Function/2
  Constant9/1 -> Math Function/1
  Math Function/1 -> Product/2
  In1/1 -> Product/1
  Product/1 -> Out1/1

== system HvsOpen/DATAPACK/dec2byte8/Subsystem1 ==
  In1 : Inport
  Constant8 : Constant  Value=power
  Constant9 : Constant  Value=2
  Math Function : Math  Operator=pow  SaturateOnIntegerOverflow=on
  Product : Product  RndMeth=Zero
  Out1 : Outport
  wires:
  Product/1 -> Out1/1
  In1/1 -> Product/1
  Math Function/1 -> Product/2
  Constant9/1 -> Math Function/1
  Constant8/1 -> Math Function/2

== system HvsOpen/DATAPACK/dec2byte8/Subsystem2 ==
  In1 : Inport
  Constant8 : Constant  Value=power
  Constant9 : Constant  Value=2
  Math Function : Math  Operator=pow  SaturateOnIntegerOverflow=on
  Product : Product  RndMeth=Zero
  Out1 : Outport
  wires:
  Constant8/1 -> Math Function/2
  Constant9/1 -> Math Function/1
  Math Function/1 -> Product/2
  In1/1 -> Product/1
  Product/1 -> Out1/1

== system HvsOpen/DATAPACK/dec2byte8/Subsystem3 ==
  In1 : Inport
  Constant8 : Constant  Value=power
  Constant9 : Constant  Value=2
  Math Function : Math  Operator=pow  SaturateOnIntegerOverflow=on
  Product : Product  RndMeth=Zero
  Out1 : Outport
  wires:
  Product/1 -> Out1/1
  In1/1 -> Product/1
  Math Function/1 -> Product/2
  Constant9/1 -> Math Function/1
  Constant8/1 -> Math Function/2

== system HvsOpen/DATAPACK/dec2byte8/Subsystem4 ==
  In1 : Inport
  Constant8 : Constant  Value=power
  Constant9 : Constant  Value=2
  Math Function : Math  Operator=pow  SaturateOnIntegerOverflow=on
  Product : Product  RndMeth=Zero
  Out1 : Outport
  wires:
  Constant8/1 -> Math Function/2
  Constant9/1 -> Math Function/1
  Math Function/1 -> Product/2
  In1/1 -> Product/1
  Product/1 -> Out1/1

== system HvsOpen/DATAPACK/dec2byte8/Subsystem5 ==
  In1 : Inport
  Constant8 : Constant  Value=power
  Constant9 : Constant  Value=2
  Math Function : Math  Operator=pow  SaturateOnIntegerOverflow=on
  Product : Product  RndMeth=Zero
  Out1 : Outport
  wires:
  Product/1 -> Out1/1
  In1/1 -> Product/1
  Math Function/1 -> Product/2
  Constant9/1 -> Math Function/1
  Constant8/1 -> Math Function/2

== system HvsOpen/DATAPACK/dec2byte8/Subsystem6 ==
  In1 : Inport
  Constant8 : Constant  Value=power
  Constant9 : Constant  Value=2
  Math Function : Math  Operator=pow  SaturateOnIntegerOverflow=on
  Product : Product  RndMeth=Zero
  Out1 : Outport
  wires:
  Constant8/1 -> Math Function/2
  Constant9/1 -> Math Function/1
  Math Function/1 -> Product/2
  In1/1 -> Product/1
  Product/1 -> Out1/1
